simulink model "simTD"  (R2015a)
settings: Solver=ode4  StartTime=0.0  StopTime=T_sim  FixedStep=Ts  RelTol=1e-3
values from neighbouring files (symbols this model uses):
  Cd = [0 0 1 0 0 0]    [Main.m]    (also in main_CG.m; main_TD.m)
  Kd_fb = Kd(:,1:nx)    [Main.m]    (also in main_CG.m; main_TD.m)
  Kd_ff = Kd(:,nx+1:end)    [Main.m]    (also in main_CG.m; main_TD.m)
  nx = size(Phi,1)    [CG_Offline.m]
  ref = 10    [Main.m]    (also in main_TC.m; main_TD.m)
  Ts = 0.01    [Main.m]    (also in main_CG.m; main_TC.m; main_TD.m)
undefined symbols (not defined in the file or in its folder): Ad, Bd, nu
settings Model: CovSFcnEnable=off  Creator=pier  LastModifiedBy=Piero
settings DebuggingCC: SolverPrmCheckMsg=warning

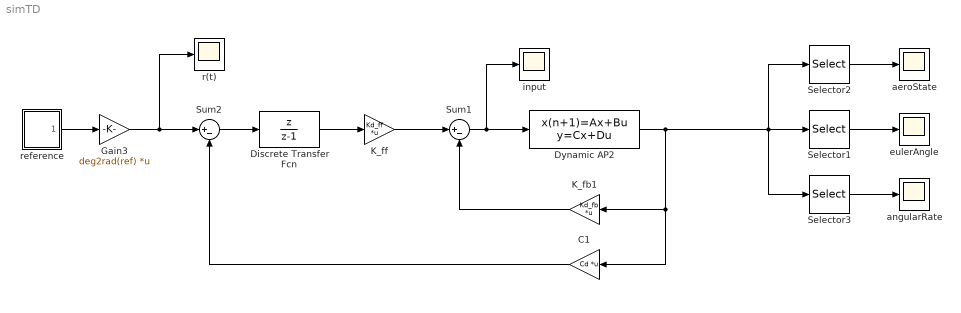
== system simTD ==
  C1 : Gain  Gain=Cd  Multiplication=Matrix(K*u)
  Discrete Transfer Fcn : DiscreteTransferFcn  Numerator=[1 0]  Denominator=[1 -1]  SampleTime=Ts
  Dynamic AP2 : DiscreteStateSpace  A=Ad  B=Bd  C=eye(nx)  D=zeros(nx,nu)  SampleTime=Ts
  Gain3 : Gain  Gain=deg2rad(ref)  Multiplication=Matrix(K*u)
  K_fb1 : Gain  Gain=Kd_fb  Multiplication=Matrix(K*u)
  K_ff : Gain  Gain=Kd_ff  Multiplication=Matrix(K*u)
  Selector1 : Selector  InputPortWidth=6  Indices=[3:4]
  Selector2 : Selector  InputPortWidth=6  Indices=[1:2]
  Selector3 : Selector  InputPortWidth=6  Indices=[5:6]
  Sum1 : Sum  Inputs=|+-
  Sum2 : Sum  Inputs=|+-
  aeroState : Scope
      settings: TimeRange=100  SaveName=sim_aeroStateTD
  angularRate : Scope
      settings: SaveName=sim_realInputTD
  eulerAngle : Scope
      settings: TimeRange=10  YMin=-0.025  YMax=0.275  SaveName=sim_eulerAnglesTD
  input : Scope
      settings: TimeRange=100  SaveName=sim_InputsTD
  r(t) : Scope
      settings: TimeRange=100  SaveName=sim_reference
  reference : Subsystem
  wires:
  reference/1(Out1) -> Gain3/1
  Gain3/1 -> Sum2/1, r(t)/1
  Selector1/1 -> eulerAngle/1
  Selector3/1 -> angularRate/1
  Selector2/1 -> aeroState/1
  Dynamic AP2/1 -> Selector3/1, Selector1/1, Selector2/1, K_fb1/1, C1/1
  Sum1/1 -> Dynamic AP2/1, input/1
  K_fb1/1 -> Sum1/2
  C1/1 -> Sum2/2
  Sum2/1 -> Discrete Transfer Fcn/1
  Discrete Transfer Fcn/1 -> K_ff/1
  K_ff/1 -> Sum1/1

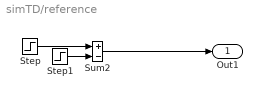
== system simTD/reference ==
  Step : Step  Time=2.5  SampleTime=0
  Step1 : Step  Time=12.5  SampleTime=0
  Sum2 : Sum  Inputs=+-
  Out1 : Outport
  wires:
  Sum2/1 -> Out1/1
  Step/1 -> Sum2/1
  Step1/1 -> Sum2/2
